simulink model "Controlador_Digital_Simulation_Lugar_das_Raizes"  (R2017a)
settings: Solver=VariableStepAuto  StartTime=0.0  StopTime=0.5  MaxStep=0.0005  RelTol=1e-5  AbsTol=1e-5
values from neighbouring files (symbols this model uses):
  Ts = 1/Fs    (= 0.00540540540541)    [Controlador_Digital_Lugar_das_Raízes.m]
undefined symbols (not defined in the file or in its folder): denc, deng, numc, numg
libraries: simulink x2
settings Model: Creator=Cleissom  LastModifiedBy=Cleissom

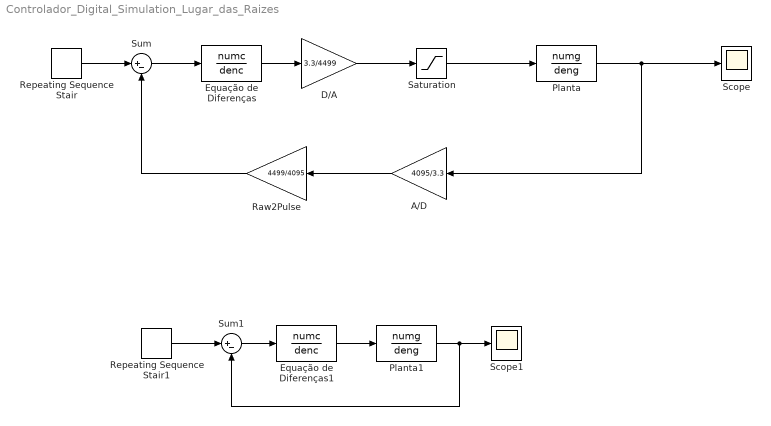
== system Controlador_Digital_Simulation_Lugar_das_Raizes ==
  A/D : Gain  Gain=4095/3.3
  D/A : Gain  Gain=3.3/4499
  Equação de Diferenças : DiscreteTransferFcn  Numerator=numc  Denominator=denc  SampleTime=Ts
  Equação de Diferenças1 : DiscreteTransferFcn  Numerator=numc  Denominator=denc  SampleTime=Ts
  Planta : TransferFcn  Numerator=numg  Denominator=deng
  Planta1 : TransferFcn  Numerator=numg  Denominator=deng
  Raw2Pulse : Gain  Gain=4499/4095
  Repeating Sequence Stair : simulink/Sources/Repeating Sequence Stair  OutValues=[1363 2045].'  tsamp=0.1  OutMin=[]  OutMax=[]  OutDataTypeStr=double  OutputDataTypeScalingMode=double  OutDataType=fixdt(0,8)  ConRadixGroup=Best Precision: Vector-wise  OutScaling=2^-12
  Repeating Sequence Stair1 : simulink/Sources/Repeating Sequence Stair  OutValues=[1 1.5].'  tsamp=0.1  OutMin=[]  OutMax=[]  OutDataTypeStr=double  OutputDataTypeScalingMode=double  OutDataType=fixdt(0,8)  ConRadixGroup=Best Precision: Vector-wise  OutScaling=2^-12
  Saturation : Saturate  UpperLimit=3.3  LowerLimit=0
  Scope : Scope
  Scope1 : Scope
  Sum : Sum  Inputs=|+-
  Sum1 : Sum  Inputs=|+-
  wires:
  Planta/1 -> Scope/1, A/D/1
  Sum/1 -> Equação de Diferenças/1
  Equação de Diferenças/1 -> D/A/1
  D/A/1 -> Saturation/1
  Raw2Pulse/1 -> Sum/2
  A/D/1 -> Raw2Pulse/1
  Repeating Sequence Stair/1 -> Sum/1
  Saturation/1 -> Planta/1
  Equação de Diferenças1/1 -> Planta1/1
  Repeating Sequence Stair1/1 -> Sum1/1
  Planta1/1 -> Scope1/1, Sum1/2
  Sum1/1 -> Equação de Diferenças1/1
